simulink model "CartPendulumPID"  (R2019a)
settings: Solver=FixedStepAuto  StartTime=0.0  StopTime=20  RelTol=1e-3
InitFcn:
  | run Initialize.m
StopFcn:
  | run Visualization.m
values from neighbouring files (symbols this model uses):
  Ts = 10*10^-3    (= 0.01)    [Initialize.m]
  x0 = [0; 0; 10*pi/180; 0]    [Initialize.m]
settings Model: Creator=visha  LastModifiedBy=visha

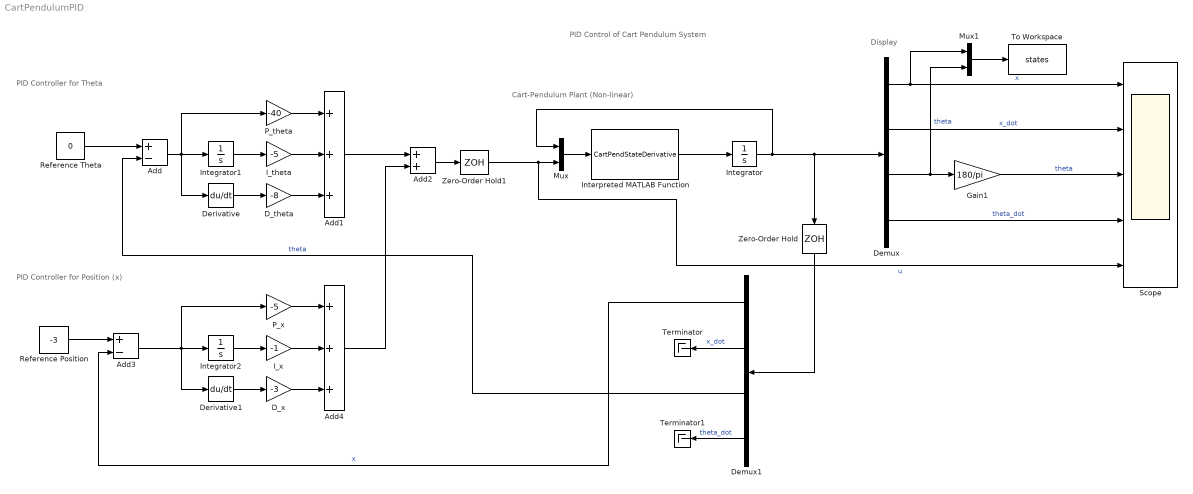
== system CartPendulumPID ==
  note: PID Control of Cart Pendulum System
  note: Display
  note: PID Controller for Theta
  note: Cart-Pendulum Plant (Non-linear)
  note: PID Controller for Position (x)
  Add : Sum  Inputs=+-
  Add1 : Sum  Inputs=+++
  Add2 : Sum
  Add3 : Sum  Inputs=+-
  Add4 : Sum  Inputs=+++
  D_theta : Gain  Gain=-8
  D_x : Gain  Gain=-3
  Demux : Demux
  Demux1 : Demux
  Derivative : Derivative
  Derivative1 : Derivative
  Gain1 : Gain  Gain=180/pi
  I_theta : Gain  Gain=-5
  I_x : Gain  Gain=-1
  Integrator : Integrator  InitialCondition=x0
  Integrator1 : Integrator
  Integrator2 : Integrator
  Interpreted MATLAB Function : MATLABFcn  MATLABFcn=CartPendStateDerivative
  Mux : Mux  Inputs=2
  Mux1 : Mux  Inputs=2
  P_theta : Gain  Gain=-40
  P_x : Gain  Gain=-5
  Reference Position : Constant  Value=-3
  Reference Theta : Constant  Value=0
  Scope : Scope  NumInputPorts=5
  Terminator : Terminator
  Terminator1 : Terminator
  To Workspace : ToWorkspace  VariableName=states  SaveFormat=Timeseries  SampleTime=-1
  Zero-Order Hold : ZeroOrderHold  SampleTime=Ts
  Zero-Order Hold1 : ZeroOrderHold  SampleTime=Ts
  wires:
  Integrator/1 -> Mux/1, Zero-Order Hold/1, Demux/1
  Interpreted MATLAB Function/1 -> Integrator/1
  Mux/1 -> Interpreted MATLAB Function/1
  Demux/4 -> Scope/4  "theta_dot"
  Demux/2 -> Scope/2  "x_dot"
  Demux/1 -> Mux1/1, Scope/1  "x"
  Demux/3 -> Gain1/1, Mux1/2  "theta"
  Mux1/1 -> To Workspace/1
  Zero-Order Hold1/1 -> Scope/5, Mux/2  "u"
  Gain1/1 -> Scope/3  "theta"
  Zero-Order Hold/1 -> Demux1/1
  Demux1/1 -> Add3/2  "x"
  Demux1/2 -> Terminator/1  "x_dot"
  Demux1/4 -> Terminator1/1  "theta_dot"
  Reference Theta/1 -> Add/1
  P_theta/1 -> Add1/1
  I_theta/1 -> Add1/2
  D_theta/1 -> Add1/3
  Add2/1 -> Zero-Order Hold1/1
  Add1/1 -> Add2/1
  Add/1 -> P_theta/1, Derivative/1, Integrator1/1
  Integrator1/1 -> I_theta/1
  Derivative/1 -> D_theta/1
  Derivative1/1 -> D_x/1
  Integrator2/1 -> I_x/1
  Add3/1 -> Integrator2/1, Derivative1/1, P_x/1
  D_x/1 -> Add4/3
  I_x/1 -> Add4/2
  P_x/1 -> Add4/1
  Reference Position/1 -> Add3/1
  Demux1/3 -> Add/2  "theta"
  Add4/1 -> Add2/2
